simulink model "Grid_modelling_Thermal_V7_ALfix_sheddable"  (R2026a)
settings: Solver=ode45  StopTime=5000  MaxStep=0.01
libraries: sl_discontinuities x10, slpidlib x10, simulink x10
(part 2 of 3)

== system Grid_modelling_Thermal_V7_ALfix_sheddable/DAB_Model_HK ==
  phase_shift : Inport
  v_left : Inport  Port=2
  v_right : Inport  Port=3
  1/2*pi*fs : Gain  Gain=1 / (2*pi*10e3)
  1/Lk : Gain  Gain=1 / 340e-6
  Abs : Abs  SaturateOnIntegerOverflow=off
  Add Constant : Bias  Bias=1  SaturateOnIntegerOverflow=off
  Constant : Constant  Value=10
  DAB_Thermal_Model : Subsystem
  Divide : Product  Inputs=*/
  Divide1 : Product  Inputs=*/
  Gain : Gain  Gain=-1/pi
  Gain1 : Gain  Gain=-1
  Max : MinMax  Function=max  Inputs=2
  Max1 : MinMax  Function=max  Inputs=2
  Product : Product
  Product1 : Product  Inputs=3
  Saturation : Saturate  UpperLimit=pi/2  LowerLimit=-pi/2
  Saturation Dynamic : sl_discontinuities/Saturation Dynamic  OutMin=[]  OutMax=[]  OutDataTypeStr=Inherit: Same as second input  OutDataType=fixdt(1, 16)  OutScaling=2^-10  DoSatur=off
  V7DERLOG_V7DER_HK : ToWorkspace  VariableName=V7DER_HK  SaveFormat=Timeseries  SampleTime=0.01
  V7LOG_V7PH_HK : ToWorkspace  VariableName=V7PH_HK  SaveFormat=Timeseries  SampleTime=0.01
  V7TJLOG_V7TJ_HK : ToWorkspace  VariableName=V7TJ_HK  SaveFormat=Timeseries  SampleTime=0.01
  deg_2_rad : Gain  Gain=pi / 180
  thermal_derater : Subsystem
  turns_ratio : Gain  Gain=24/15
  i_dab_i : Outport
  i_dab_j : Outport  Port=2
  dab_k : Outport  Port=3
  Temp_Junction : Outport  Port=4
  Temp_HeatSink : Outport  Port=5
  wires:
  Constant/1 -> Max/2, Max1/2
  Add Constant/1 -> Product1/2
  Divide/1 -> Gain1/1
  Max1/1 -> Divide1/2
  Gain1/1 -> i_dab_i/1
  Divide1/1 -> i_dab_j/1
  Saturation Dynamic/1 -> DAB_Thermal_Model/1(P_ij), Divide1/1, Divide/1
  Saturation/1 -> Product1/1, Abs/1
  1/2*pi*fs/1 -> 1/Lk/1
  phase_shift/1 -> deg_2_rad/1, V7LOG_V7PH_HK/1
  Gain/1 -> Add Constant/1
  1/Lk/1 -> dab_k/1, Product1/3
  Product/1 -> turns_ratio/1
  turns_ratio/1 -> 1/2*pi*fs/1
  Abs/1 -> Gain/1
  deg_2_rad/1 -> Saturation/1
  Max/1 -> Divide/2
  v_right/1 -> DAB_Thermal_Model/3(Vb), Product/2, Max1/1
  v_left/1 -> DAB_Thermal_Model/2(Va), Max/1, Product/1
  Product1/1 -> Saturation Dynamic/2  "P_ij"
  DAB_Thermal_Model/1(T_j) -> thermal_derater/1(Tj), Temp_Junction/1, V7TJLOG_V7TJ_HK/1
  DAB_Thermal_Model/2(T_h) -> Temp_HeatSink/1
  thermal_derater/1(derate_pos) -> Saturation Dynamic/1, V7DERLOG_V7DER_HK/1
  thermal_derater/2(derate_neg) -> Saturation Dynamic/3

== system Grid_modelling_Thermal_V7_ALfix_sheddable/DAB_Model_KL ==
  phase_shift : Inport
  v_left : Inport  Port=2
  v_right : Inport  Port=3
  1/2*pi*fs : Gain  Gain=1 / (2*pi*10e3)
  1/Lk : Gain  Gain=1 / 340e-6
  Abs : Abs  SaturateOnIntegerOverflow=off
  Add Constant : Bias  Bias=1  SaturateOnIntegerOverflow=off
  Constant : Constant  Value=10
  DAB_Thermal_Model : Subsystem
  Divide : Product  Inputs=*/
  Divide1 : Product  Inputs=*/
  Gain : Gain  Gain=-1/pi
  Gain1 : Gain  Gain=-1
  Max : MinMax  Function=max  Inputs=2
  Max1 : MinMax  Function=max  Inputs=2
  Product : Product
  Product1 : Product  Inputs=3
  Saturation : Saturate  UpperLimit=pi/2  LowerLimit=-pi/2
  Saturation Dynamic : sl_discontinuities/Saturation Dynamic  OutMin=[]  OutMax=[]  OutDataTypeStr=Inherit: Same as second input  OutDataType=fixdt(1, 16)  OutScaling=2^-10  DoSatur=off
  V7DERLOG_V7DER_KL : ToWorkspace  VariableName=V7DER_KL  SaveFormat=Timeseries  SampleTime=0.01
  V7LOG_V7PH_KL : ToWorkspace  VariableName=V7PH_KL  SaveFormat=Timeseries  SampleTime=0.01
  V7TJLOG_V7TJ_KL : ToWorkspace  VariableName=V7TJ_KL  SaveFormat=Timeseries  SampleTime=0.01
  deg_2_rad : Gain  Gain=pi / 180
  thermal_derater : Subsystem
  turns_ratio : Gain  Gain=24/15
  i_dab_i : Outport
  i_dab_j : Outport  Port=2
  dab_k : Outport  Port=3
  Temp_Junction : Outport  Port=4
  Temp_HeatSink : Outport  Port=5
  wires:
  Constant/1 -> Max/2, Max1/2
  Add Constant/1 -> Product1/2
  Divide/1 -> Gain1/1
  Max1/1 -> Divide1/2
  Gain1/1 -> i_dab_i/1
  Divide1/1 -> i_dab_j/1
  Saturation Dynamic/1 -> DAB_Thermal_Model/1(P_ij), Divide1/1, Divide/1
  Saturation/1 -> Product1/1, Abs/1
  1/2*pi*fs/1 -> 1/Lk/1
  phase_shift/1 -> deg_2_rad/1, V7LOG_V7PH_KL/1
  Gain/1 -> Add Constant/1
  1/Lk/1 -> dab_k/1, Product1/3
  Product/1 -> turns_ratio/1
  turns_ratio/1 -> 1/2*pi*fs/1
  Abs/1 -> Gain/1
  deg_2_rad/1 -> Saturation/1
  Max/1 -> Divide/2
  v_right/1 -> DAB_Thermal_Model/3(Vb), Product/2, Max1/1
  v_left/1 -> DAB_Thermal_Model/2(Va), Max/1, Product/1
  Product1/1 -> Saturation Dynamic/2  "P_ij"
  DAB_Thermal_Model/1(T_j) -> thermal_derater/1(Tj), Temp_Junction/1, V7TJLOG_V7TJ_KL/1
  DAB_Thermal_Model/2(T_h) -> Temp_HeatSink/1
  thermal_derater/1(derate_pos) -> Saturation Dynamic/1, V7DERLOG_V7DER_KL/1
  thermal_derater/2(derate_neg) -> Saturation Dynamic/3

== system Grid_modelling_Thermal_V7_ALfix_sheddable/source_bus_model_A ==
  Pload : Inport
  i_dab_1 : Inport  Port=2
  i_dab_2 : Inport  Port=3
  1/C_bus : Gain  Gain=1/0.01
  1/Rsrc_k : Gain  Gain=1/(0.32*1)
  Add : Sum  Inputs=+-++
  Bus_Bar_Thermal_Model : Subsystem
  Constant : Constant  Value=0
  Divide : Product  Inputs=*/
  Divide1 : Product  Inputs=*/
  I_max : Constant  Value=125
  Integrator : Integrator  InitialCondition=800  LimitOutput=on  LowerSaturationLimit=0
  Max : MinMax  Function=max  Inputs=2
  Max1 : MinMax  Function=max  Inputs=2
  Max2 : MinMax  Function=max  Inputs=2
  Min : MinMax  Inputs=2
  Min1 : MinMax  Inputs=2
  P_max : Constant  Value=100e3
  Product : Product
  Subtract : Sum  Inputs=+-
  V_th_k : Constant  Value=800
  div_by_zero_protect : Constant  Value=10
  div_by_zero_protect1 : Constant  Value=10
  V_bus : Outport
  Bus_Power : Outport  Port=2
  Temp_bus : Outport  Port=3
  wires:
  Max2/1 -> Divide1/2
  Divide/1 -> Min1/2  "i_pmax_k"
  1/Rsrc_k/1 -> Max/1  "i_th_k"
  Min/1 -> Min1/1  "i_lim_k"
  Subtract/1 -> 1/Rsrc_k/1
  Add/1 -> 1/C_bus/1
  1/C_bus/1 -> Integrator/1
  Integrator/1 -> Product/1, V_bus/1, Max2/1, Max1/1, Subtract/2
  Divide1/1 -> Add/2
  V_th_k/1 -> Subtract/1
  Pload/1 -> Divide1/1
  Constant/1 -> Max/2
  Max/1 -> Min/1
  i_dab_1/1 -> Add/3
  I_max/1 -> Min/2
  Min1/1 -> Add/1, Bus_Bar_Thermal_Model/1(i_src_k), Product/2  "i_src_k"
  P_max/1 -> Divide/1
  Max1/1 -> Divide/2
  i_dab_2/1 -> Add/4
  div_by_zero_protect1/1 -> Max2/2
  div_by_zero_protect/1 -> Max1/2
  Product/1 -> Bus_Power/1
  Bus_Bar_Thermal_Model/1(T_bus) -> Temp_bus/1

== system Grid_modelling_Thermal_V7_ALfix_sheddable/source_bus_model_B ==
  Pload : Inport
  i_dab_1 : Inport  Port=2
  i_dab_2 : Inport  Port=3
  1/C_bus : Gain  Gain=1/0.01
  Add : Sum  Inputs=+-++
  Bus_Bar_Thermal_Model : Subsystem
  Constant : Constant  Value=0
  Divide : Product  Inputs=*/
  Divide1 : Product  Inputs=*/
  I_max : Constant  Value=125
  Integrator : Integrator  InitialCondition=800  LimitOutput=on  LowerSaturationLimit=0
  Max : MinMax  Function=max  Inputs=2
  Max1 : MinMax  Function=max  Inputs=2
  Max2 : MinMax  Function=max  Inputs=2
  Min : MinMax  Inputs=2
  Min1 : MinMax  Inputs=2
  P_max : Constant  Value=100e3
  Product : Product
  Product1 : Product
  Step : Step  Time=1000  InitialValue=1 / (0.32*1)  FinalValue=1 / (0.32*1)  SampleTime=0
  Subtract : Sum  Inputs=+-
  V_th_k : Constant  Value=800
  div_by_zero_protect : Constant  Value=10
  div_by_zero_protect1 : Constant  Value=10
  V_bus : Outport
  Bus_Power : Outport  Port=2
  Temp_bus : Outport  Port=3
  wires:
  Max2/1 -> Divide1/2
  Divide/1 -> Min1/2  "i_pmax_k"
  Product1/1 -> Max/1  "i_th_k"
  Min/1 -> Min1/1  "i_lim_k"
  Subtract/1 -> Product1/2
  Add/1 -> 1/C_bus/1
  1/C_bus/1 -> Integrator/1
  Divide1/1 -> Add/2
  V_th_k/1 -> Subtract/1
  Pload/1 -> Divide1/1
  Constant/1 -> Max/2
  Max/1 -> Min/1
  i_dab_1/1 -> Add/3
  I_max/1 -> Min/2
  P_max/1 -> Divide/1
  Max1/1 -> Divide/2
  i_dab_2/1 -> Add/4
  div_by_zero_protect1/1 -> Max2/2
  div_by_zero_protect/1 -> Max1/2
  Integrator/1 -> Product/1, V_bus/1, Max2/1, Max1/1, Subtract/2
  Product/1 -> Bus_Power/1
  Min1/1 -> Bus_Bar_Thermal_Model/1(i_src_k), Product/2, Add/1  "i_src_k"
  Bus_Bar_Thermal_Model/1(T_bus) -> Temp_bus/1
  Step/1 -> Product1/1

== system Grid_modelling_Thermal_V7_ALfix_sheddable/source_bus_model_C ==
  Pload : Inport
  i_dab_1 : Inport  Port=2
  i_dab_2 : Inport  Port=3
  1/C_bus : Gain  Gain=1/0.01
  Add : Sum  Inputs=+-++
  Bus_Bar_Thermal_Model : Subsystem
  Constant : Constant  Value=0
  Divide : Product  Inputs=*/
  Divide1 : Product  Inputs=*/
  I_max : Constant  Value=125
  Integrator : Integrator  InitialCondition=800  LimitOutput=on  LowerSaturationLimit=0
  Max : MinMax  Function=max  Inputs=2
  Max1 : MinMax  Function=max  Inputs=2
  Max2 : MinMax  Function=max  Inputs=2
  Min : MinMax  Inputs=2
  Min1 : MinMax  Inputs=2
  P_max : Constant  Value=100e3
  Product : Product
  Product1 : Product
  Step : Step  Time=2250  InitialValue=1 / (0.32*1)  FinalValue=1 / (0.32*1)  SampleTime=0
  Subtract : Sum  Inputs=+-
  V_th_k : Constant  Value=800
  div_by_zero_protect : Constant  Value=10
  div_by_zero_protect1 : Constant  Value=10
  V_bus : Outport
  Bus_Power : Outport  Port=2
  Temp_bus : Outport  Port=3
  wires:
  Max2/1 -> Divide1/2
  Divide/1 -> Min1/2  "i_pmax_k"
  Product1/1 -> Max/1  "i_th_k"
  Min/1 -> Min1/1  "i_lim_k"
  Subtract/1 -> Product1/2
  Add/1 -> 1/C_bus/1
  1/C_bus/1 -> Integrator/1
  Divide1/1 -> Add/2
  V_th_k/1 -> Subtract/1
  Pload/1 -> Divide1/1
  Constant/1 -> Max/2
  Max/1 -> Min/1
  i_dab_1/1 -> Add/3
  I_max/1 -> Min/2
  P_max/1 -> Divide/1
  Max1/1 -> Divide/2
  i_dab_2/1 -> Add/4
  div_by_zero_protect1/1 -> Max2/2
  div_by_zero_protect/1 -> Max1/2
  Integrator/1 -> Product/1, V_bus/1, Max2/1, Max1/1, Subtract/2
  Product/1 -> Bus_Power/1
  Min1/1 -> Bus_Bar_Thermal_Model/1(i_src_k), Product/2, Add/1  "i_src_k"
  Bus_Bar_Thermal_Model/1(T_bus) -> Temp_bus/1
  Step/1 -> Product1/1

== system Grid_modelling_Thermal_V7_ALfix_sheddable/source_bus_model_D ==
  Pload : Inport
  i_dab_1 : Inport  Port=2
  i_dab_2 : Inport  Port=3
  1/C_bus : Gain  Gain=1/0.01
  1/Rsrc_k : Gain  Gain=1/(0.32*1)
  Add : Sum  Inputs=+-++
  Bus_Bar_Thermal_Model : Subsystem
  Constant : Constant  Value=0
  Divide : Product  Inputs=*/
  Divide1 : Product  Inputs=*/
  I_max : Constant  Value=125
  Integrator : Integrator  InitialCondition=800  LimitOutput=on  LowerSaturationLimit=0
  Max : MinMax  Function=max  Inputs=2
  Max1 : MinMax  Function=max  Inputs=2
  Max2 : MinMax  Function=max  Inputs=2
  Min : MinMax  Inputs=2
  Min1 : MinMax  Inputs=2
  P_max : Constant  Value=100e3
  Product : Product
  Subtract : Sum  Inputs=+-
  V_th_k : Constant  Value=800
  div_by_zero_protect : Constant  Value=10
  div_by_zero_protect1 : Constant  Value=10
  V_bus : Outport
  Bus_Power : Outport  Port=2
  Temp_bus : Outport  Port=3
  wires:
  Max2/1 -> Divide1/2
  Divide/1 -> Min1/2  "i_pmax_k"
  1/Rsrc_k/1 -> Max/1  "i_th_k"
  Min/1 -> Min1/1  "i_lim_k"
  Subtract/1 -> 1/Rsrc_k/1
  Add/1 -> 1/C_bus/1
  1/C_bus/1 -> Integrator/1
  Divide1/1 -> Add/2
  V_th_k/1 -> Subtract/1
  Pload/1 -> Divide1/1
  Constant/1 -> Max/2
  Max/1 -> Min/1
  i_dab_1/1 -> Add/3
  I_max/1 -> Min/2
  P_max/1 -> Divide/1
  Max1/1 -> Divide/2
  i_dab_2/1 -> Add/4
  div_by_zero_protect1/1 -> Max2/2
  div_by_zero_protect/1 -> Max1/2
  Integrator/1 -> Product/1, V_bus/1, Max2/1, Max1/1, Subtract/2
  Product/1 -> Bus_Power/1
  Min1/1 -> Bus_Bar_Thermal_Model/1(i_src_k), Product/2, Add/1  "i_src_k"
  Bus_Bar_Thermal_Model/1(T_bus) -> Temp_bus/1

== system Grid_modelling_Thermal_V7_ALfix_sheddable/source_bus_model_E ==
  Pload : Inport
  i_dab_1 : Inport  Port=2
  i_dab_2 : Inport  Port=3
  1/C_bus : Gain  Gain=1/0.01
  Add : Sum  Inputs=+-++
  Bus_Bar_Thermal_Model : Subsystem
  Constant : Constant  Value=0
  Divide : Product  Inputs=*/
  Divide1 : Product  Inputs=*/
  I_max : Constant  Value=125
  Integrator : Integrator  InitialCondition=800  LimitOutput=on  LowerSaturationLimit=0
  Max : MinMax  Function=max  Inputs=2
  Max1 : MinMax  Function=max  Inputs=2
  Max2 : MinMax  Function=max  Inputs=2
  Min : MinMax  Inputs=2
  Min1 : MinMax  Inputs=2
  P_max : Constant  Value=70e3
  Product : Product
  Product1 : Product
  Step : Step  Time=1500  InitialValue=1 / (0.32*1)  FinalValue=1 / (0.32*2)  SampleTime=0
  Subtract : Sum  Inputs=+-
  V_th_k : Constant  Value=800
  div_by_zero_protect : Constant  Value=10
  div_by_zero_protect1 : Constant  Value=10
  V_bus : Outport
  Bus_Power : Outport  Port=2
  Temp_bus : Outport  Port=3
  wires:
  Max2/1 -> Divide1/2
  Divide/1 -> Min1/2  "i_pmax_k"
  Product1/1 -> Max/1  "i_th_k"
  Min/1 -> Min1/1  "i_lim_k"
  Subtract/1 -> Product1/2
  Add/1 -> 1/C_bus/1
  1/C_bus/1 -> Integrator/1
  Divide1/1 -> Add/2
  V_th_k/1 -> Subtract/1
  Pload/1 -> Divide1/1
  Constant/1 -> Max/2
  Max/1 -> Min/1
  i_dab_1/1 -> Add/3
  I_max/1 -> Min/2
  P_max/1 -> Divide/1
  Max1/1 -> Divide/2
  i_dab_2/1 -> Add/4
  div_by_zero_protect1/1 -> Max2/2
  div_by_zero_protect/1 -> Max1/2
  Integrator/1 -> Product/1, V_bus/1, Max2/1, Max1/1, Subtract/2
  Product/1 -> Bus_Power/1
  Min1/1 -> Bus_Bar_Thermal_Model/1(i_src_k), Product/2, Add/1  "i_src_k"
  Bus_Bar_Thermal_Model/1(T_bus) -> Temp_bus/1
  Step/1 -> Product1/1

== system Grid_modelling_Thermal_V7_ALfix_sheddable/source_bus_model_F ==
  Pload : Inport
  i_dab_1 : Inport  Port=2
  i_dab_2 : Inport  Port=3
  1/C_bus : Gain  Gain=1/0.01
  Add : Sum  Inputs=+-++
  Bus_Bar_Thermal_Model : Subsystem
  Constant : Constant  Value=0
  Divide : Product  Inputs=*/
  Divide1 : Product  Inputs=*/
  I_max : Constant  Value=125
  Integrator : Integrator  InitialCondition=800  LimitOutput=on  LowerSaturationLimit=0
  Max : MinMax  Function=max  Inputs=2
  Max1 : MinMax  Function=max  Inputs=2
  Max2 : MinMax  Function=max  Inputs=2
  Min : MinMax  Inputs=2
  Min1 : MinMax  Inputs=2
  P_max : Constant  Value=70e3
  Product : Product
  Product1 : Product
  Step : Step  Time=1250  InitialValue=1 / (0.32*1)  FinalValue=1 / (0.32*2)  SampleTime=0
  Subtract : Sum  Inputs=+-
  V_th_k : Constant  Value=800
  div_by_zero_protect : Constant  Value=10
  div_by_zero_protect1 : Constant  Value=10
  V_bus : Outport
  Bus_Power : Outport  Port=2
  Temp_bus : Outport  Port=3
  wires:
  Max2/1 -> Divide1/2
  Divide/1 -> Min1/2  "i_pmax_k"
  Product1/1 -> Max/1  "i_th_k"
  Min/1 -> Min1/1  "i_lim_k"
  Subtract/1 -> Product1/2
  Add/1 -> 1/C_bus/1
  1/C_bus/1 -> Integrator/1
  Divide1/1 -> Add/2
  V_th_k/1 -> Subtract/1
  Pload/1 -> Divide1/1
  Constant/1 -> Max/2
  Max/1 -> Min/1
  i_dab_1/1 -> Add/3
  I_max/1 -> Min/2
  P_max/1 -> Divide/1
  Max1/1 -> Divide/2
  i_dab_2/1 -> Add/4
  div_by_zero_protect1/1 -> Max2/2
  div_by_zero_protect/1 -> Max1/2
  Integrator/1 -> Product/1, V_bus/1, Max2/1, Max1/1, Subtract/2
  Product/1 -> Bus_Power/1
  Min1/1 -> Bus_Bar_Thermal_Model/1(i_src_k), Product/2, Add/1  "i_src_k"
  Bus_Bar_Thermal_Model/1(T_bus) -> Temp_bus/1
  Step/1 -> Product1/1

== system Grid_modelling_Thermal_V7_ALfix_sheddable/source_bus_model_G ==
  Pload : Inport
  i_dab_1 : Inport  Port=2
  i_dab_2 : Inport  Port=3
  1/C_bus : Gain  Gain=1/0.01
  1/Rsrc_k : Gain  Gain=1/(0.32*1)
  Add : Sum  Inputs=+-++
  Bus_Bar_Thermal_Model : Subsystem
  Constant : Constant  Value=0
  Divide : Product  Inputs=*/
  Divide1 : Product  Inputs=*/
  I_max : Constant  Value=125
  Integrator : Integrator  InitialCondition=800  LimitOutput=on  LowerSaturationLimit=0
  Max : MinMax  Function=max  Inputs=2
  Max1 : MinMax  Function=max  Inputs=2
  Max2 : MinMax  Function=max  Inputs=2
  Min : MinMax  Inputs=2
  Min1 : MinMax  Inputs=2
  P_max : Constant  Value=100e3
  Product : Product
  Subtract : Sum  Inputs=+-
  V_th_k : Constant  Value=800
  div_by_zero_protect : Constant  Value=10
  div_by_zero_protect1 : Constant  Value=10
  V_bus : Outport
  Bus_Power : Outport  Port=2
  Temp_bus : Outport  Port=3
  wires:
  Max2/1 -> Divide1/2
  Divide/1 -> Min1/2  "i_pmax_k"
  1/Rsrc_k/1 -> Max/1  "i_th_k"
  Min/1 -> Min1/1  "i_lim_k"
  Subtract/1 -> 1/Rsrc_k/1
  Add/1 -> 1/C_bus/1
  1/C_bus/1 -> Integrator/1
  Divide1/1 -> Add/2
  V_th_k/1 -> Subtract/1
  Pload/1 -> Divide1/1
  Constant/1 -> Max/2
  Max/1 -> Min/1
  i_dab_1/1 -> Add/3
  I_max/1 -> Min/2
  P_max/1 -> Divide/1
  Max1/1 -> Divide/2
  i_dab_2/1 -> Add/4
  div_by_zero_protect1/1 -> Max2/2
  div_by_zero_protect/1 -> Max1/2
  Integrator/1 -> Product/1, V_bus/1, Max2/1, Max1/1, Subtract/2
  Product/1 -> Bus_Power/1
  Min1/1 -> Bus_Bar_Thermal_Model/1(i_src_k), Product/2, Add/1  "i_src_k"
  Bus_Bar_Thermal_Model/1(T_bus) -> Temp_bus/1

== system Grid_modelling_Thermal_V7_ALfix_sheddable/source_bus_model_H ==
  Pload : Inport
  i_dab_1 : Inport  Port=2
  i_dab_2 : Inport  Port=3
  1/C_bus : Gain  Gain=1/0.01
  1/Rsrc_k : Gain  Gain=1/(0.32*1)
  Add : Sum  Inputs=+-++
  Bus_Bar_Thermal_Model : Subsystem
  Constant : Constant  Value=0
  Divide : Product  Inputs=*/
  Divide1 : Product  Inputs=*/
  I_max : Constant  Value=125
  Integrator : Integrator  InitialCondition=800  LimitOutput=on  LowerSaturationLimit=0
  Max : MinMax  Function=max  Inputs=2
  Max1 : MinMax  Function=max  Inputs=2
  Max2 : MinMax  Function=max  Inputs=2
  Min : MinMax  Inputs=2
  Min1 : MinMax  Inputs=2
  P_max : Constant  Value=100e3
  Product : Product
  Subtract : Sum  Inputs=+-
  V_th_k : Constant  Value=800
  div_by_zero_protect : Constant  Value=10
  div_by_zero_protect1 : Constant  Value=10
  V_bus : Outport
  Bus_Power : Outport  Port=2
  Temp_bus : Outport  Port=3
  wires:
  Max2/1 -> Divide1/2
  Divide/1 -> Min1/2  "i_pmax_k"
  1/Rsrc_k/1 -> Max/1  "i_th_k"
  Min/1 -> Min1/1  "i_lim_k"
  Subtract/1 -> 1/Rsrc_k/1
  Add/1 -> 1/C_bus/1
  1/C_bus/1 -> Integrator/1
  Divide1/1 -> Add/2
  V_th_k/1 -> Subtract/1
  Pload/1 -> Divide1/1
  Constant/1 -> Max/2
  Max/1 -> Min/1
  i_dab_1/1 -> Add/3
  I_max/1 -> Min/2
  P_max/1 -> Divide/1
  Max1/1 -> Divide/2
  i_dab_2/1 -> Add/4
  div_by_zero_protect1/1 -> Max2/2
  div_by_zero_protect/1 -> Max1/2
  Integrator/1 -> Product/1, V_bus/1, Max2/1, Max1/1, Subtract/2
  Product/1 -> Bus_Power/1
  Min1/1 -> Bus_Bar_Thermal_Model/1(i_src_k), Product/2, Add/1  "i_src_k"
  Bus_Bar_Thermal_Model/1(T_bus) -> Temp_bus/1

== system Grid_modelling_Thermal_V7_ALfix_sheddable/source_bus_model_K ==
  Pload : Inport
  i_dab_1 : Inport  Port=2
  i_dab_2 : Inport  Port=3
  1/C_bus : Gain  Gain=1/0.01
  1/Rsrc_k : Gain  Gain=1/(0.32*1)
  Add : Sum  Inputs=+-++
  Bus_Bar_Thermal_Model : Subsystem
  Constant : Constant  Value=0
  Divide : Product  Inputs=*/
  Divide1 : Product  Inputs=*/
  I_max : Constant  Value=125
  Integrator : Integrator  InitialCondition=800  LimitOutput=on  LowerSaturationLimit=0
  Max : MinMax  Function=max  Inputs=2
  Max1 : MinMax  Function=max  Inputs=2
  Max2 : MinMax  Function=max  Inputs=2
  Min : MinMax  Inputs=2
  Min1 : MinMax  Inputs=2
  P_max : Constant  Value=100e3
  Product : Product
  Subtract : Sum  Inputs=+-
  V_th_k : Constant  Value=800
  div_by_zero_protect : Constant  Value=10
  div_by_zero_protect1 : Constant  Value=10
  V_bus : Outport
  Bus_Power : Outport  Port=2
  Temp_bus : Outport  Port=3
  wires:
  Max2/1 -> Divide1/2
  Divide/1 -> Min1/2  "i_pmax_k"
  1/Rsrc_k/1 -> Max/1  "i_th_k"
  Min/1 -> Min1/1  "i_lim_k"
  Subtract/1 -> 1/Rsrc_k/1
  Add/1 -> 1/C_bus/1
  1/C_bus/1 -> Integrator/1
  Divide1/1 -> Add/2
  V_th_k/1 -> Subtract/1
  Pload/1 -> Divide1/1
  Constant/1 -> Max/2
  Max/1 -> Min/1
  i_dab_1/1 -> Add/3
  I_max/1 -> Min/2
  P_max/1 -> Divide/1
  Max1/1 -> Divide/2
  i_dab_2/1 -> Add/4
  div_by_zero_protect1/1 -> Max2/2
  div_by_zero_protect/1 -> Max1/2
  Integrator/1 -> Product/1, V_bus/1, Max2/1, Max1/1, Subtract/2
  Product/1 -> Bus_Power/1
  Min1/1 -> Bus_Bar_Thermal_Model/1(i_src_k), Product/2, Add/1  "i_src_k"
  Bus_Bar_Thermal_Model/1(T_bus) -> Temp_bus/1

== system Grid_modelling_Thermal_V7_ALfix_sheddable/source_bus_model_L ==
  Pload : Inport
  i_dab_1 : Inport  Port=2
  i_dab_2 : Inport  Port=3
  1/C_bus : Gain  Gain=1/0.01
  1/Rsrc_k : Gain  Gain=1/(0.32*1)
  Add : Sum  Inputs=+-++
  Bus_Bar_Thermal_Model : Subsystem
  Constant : Constant  Value=0
  Divide : Product  Inputs=*/
  Divide1 : Product  Inputs=*/
  I_max : Constant  Value=125
  Integrator : Integrator  InitialCondition=800  LimitOutput=on  LowerSaturationLimit=0
  Max : MinMax  Function=max  Inputs=2
  Max1 : MinMax  Function=max  Inputs=2
  Max2 : MinMax  Function=max  Inputs=2
  Min : MinMax  Inputs=2
  Min1 : MinMax  Inputs=2
  P_max : Constant  Value=100e3
  Product : Product
  Subtract : Sum  Inputs=+-
  V_th_k : Constant  Value=800
  div_by_zero_protect : Constant  Value=10
  div_by_zero_protect1 : Constant  Value=10
  V_bus : Outport
  Bus_Power : Outport  Port=2
  Temp_bus : Outport  Port=3
  wires:
  Max2/1 -> Divide1/2
  Divide/1 -> Min1/2  "i_pmax_k"
  1/Rsrc_k/1 -> Max/1  "i_th_k"
  Min/1 -> Min1/1  "i_lim_k"
  Subtract/1 -> 1/Rsrc_k/1
  Add/1 -> 1/C_bus/1
  1/C_bus/1 -> Integrator/1
  Divide1/1 -> Add/2
  V_th_k/1 -> Subtract/1
  Pload/1 -> Divide1/1
  Constant/1 -> Max/2
  Max/1 -> Min/1
  i_dab_1/1 -> Add/3
  I_max/1 -> Min/2
  P_max/1 -> Divide/1
  Max1/1 -> Divide/2
  i_dab_2/1 -> Add/4
  div_by_zero_protect1/1 -> Max2/2
  div_by_zero_protect/1 -> Max1/2
  Integrator/1 -> Product/1, V_bus/1, Max2/1, Max1/1, Subtract/2
  Product/1 -> Bus_Power/1
  Min1/1 -> Bus_Bar_Thermal_Model/1(i_src_k), Product/2, Add/1  "i_src_k"
  Bus_Bar_Thermal_Model/1(T_bus) -> Temp_bus/1

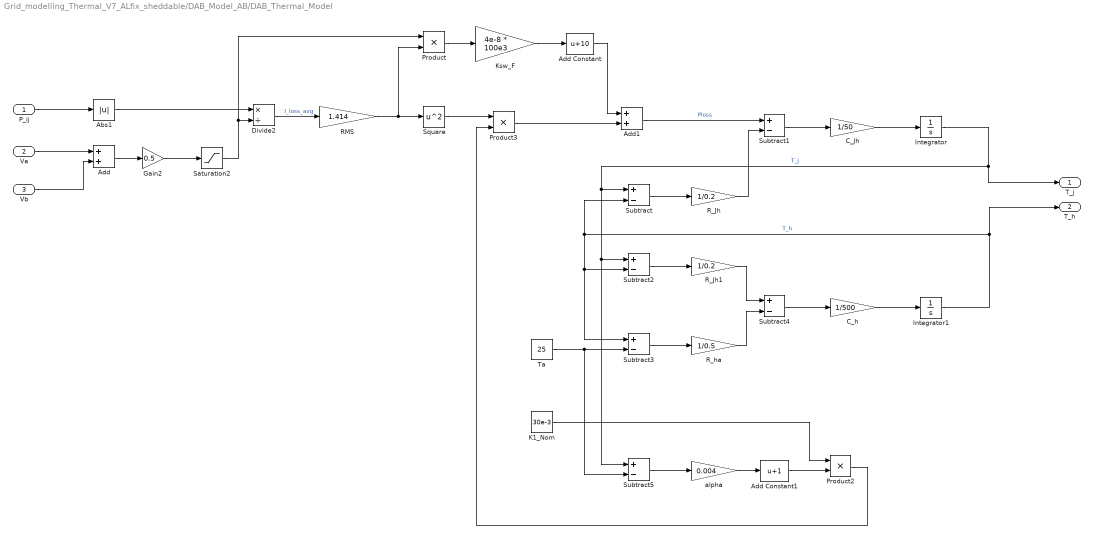
== system Grid_modelling_Thermal_V7_ALfix_sheddable/DAB_Model_AB/DAB_Thermal_Model ==
  P_ij : Inport
  Va : Inport  Port=2
  Vb : Inport  Port=3
  Abs1 : Abs  SaturateOnIntegerOverflow=off
  Add : Sum
  Add Constant : Bias  Bias=10  SaturateOnIntegerOverflow=off
  Add Constant1 : Bias  Bias=1  SaturateOnIntegerOverflow=off
  Add1 : Sum
  C_Jh : Gain  Gain=1/50
  C_h : Gain  Gain=1/500
  Divide2 : Product  Inputs=*/
  Gain2 : Gain  Gain=0.5
  Integrator : Integrator  InitialCondition=25
  Integrator1 : Integrator  InitialCondition=25
  K1_Nom : Constant  Value=30e-3
  Ksw_F : Gain  Gain=4e-8 * 100e3
  Product : Product
  Product2 : Product
  Product3 : Product
  RMS : Gain  Gain=1.414
  R_Jh : Gain  Gain=1/0.2
  R_Jh1 : Gain  Gain=1/0.2
  R_ha : Gain  Gain=1/0.5
  Saturation2 : Saturate  UpperLimit=inf  LowerLimit=1e-3
  Square : Math  Operator=square
  Subtract{,1..5} (6 alike) : Sum  Inputs=+-
  Ta : Constant  Value=25
  alpha : Gain  Gain=0.004
  T_j : Outport
  T_h : Outport  Port=2
  wires:
  Integrator/1 -> T_j/1, Subtract5/1, Subtract2/1, Subtract/1  "T_j"
  Add1/1 -> Subtract1/1  "Ploss"
  R_ha/1 -> Subtract4/2
  Gain2/1 -> Saturation2/1
  Va/1 -> Add/1
  Integrator1/1 -> T_h/1, Subtract/2, Subtract3/1, Subtract2/2  "T_h"
  R_Jh/1 -> Subtract1/2
  Add/1 -> Gain2/1
  Subtract5/1 -> alpha/1
  Subtract1/1 -> C_Jh/1
  C_h/1 -> Integrator1/1
  Divide2/1 -> RMS/1  "I_loss_avg"
  Product3/1 -> Add1/2
  P_ij/1 -> Abs1/1
  Subtract2/1 -> R_Jh1/1
  alpha/1 -> Add Constant1/1
  Product2/1 -> Product3/2
  C_Jh/1 -> Integrator/1
  Ta/1 -> Subtract5/2, Subtract3/2
  Saturation2/1 -> Product/1, Divide2/2
  R_Jh1/1 -> Subtract4/1
  Subtract/1 -> R_Jh/1
  Abs1/1 -> Divide2/1
  Subtract4/1 -> C_h/1
  Subtract3/1 -> R_ha/1
  Add Constant1/1 -> Product2/2
  Vb/1 -> Add/2
  K1_Nom/1 -> Product2/1
  Square/1 -> Product3/1
  RMS/1 -> Product/2, Square/1
  Product/1 -> Ksw_F/1
  Ksw_F/1 -> Add Constant/1
  Add Constant/1 -> Add1/1

== system Grid_modelling_Thermal_V7_ALfix_sheddable/DAB_Model_AB/thermal_derater ==
  Tj : Inport
  Gain : Gain  Gain=-1
  Gain2 : Gain  Gain=100e3
  If : If  IfExpression=u1 < 125  ElseIfExpressions=u1 > 125 & u1 < 175, u1 > 175  ShowElse=off
  If Action Subsystem : Subsystem  TreatAsAtomicUnit=on
  If Action Subsystem1 : Subsystem  TreatAsAtomicUnit=on
  If Action Subsystem2 : Subsystem  TreatAsAtomicUnit=on
  Merge : Merge  Inputs=3
  Saturation2 : Saturate  UpperLimit=1  LowerLimit=0
  Scope : Scope
      settings: ActiveDisplayYMinimum=0.36463  ActiveDisplayYMaximum=1.0706  DataLoggingVariableName=ScopeData2
  derate_pos : Outport
  derate_neg : Outport  Port=2
  wires:
  If/1 -> If Action Subsystem/Action
  Tj/1 -> If/1, If Action Subsystem1/1(Tj)
  If/3 -> If Action Subsystem2/Action
  If Action Subsystem2/1(Out1) -> Merge/3
  If Action Subsystem1/1(Out1) -> Merge/2
  Merge/1 -> Saturation2/1
  If Action Subsystem/1(Out1) -> Merge/1
  Gain2/1 -> derate_pos/1, Gain/1
  Saturation2/1 -> Scope/1, Gain2/1  "DAB_AB_derate_factor"
  Gain/1 -> derate_neg/1
  If/2 -> If Action Subsystem1/Action

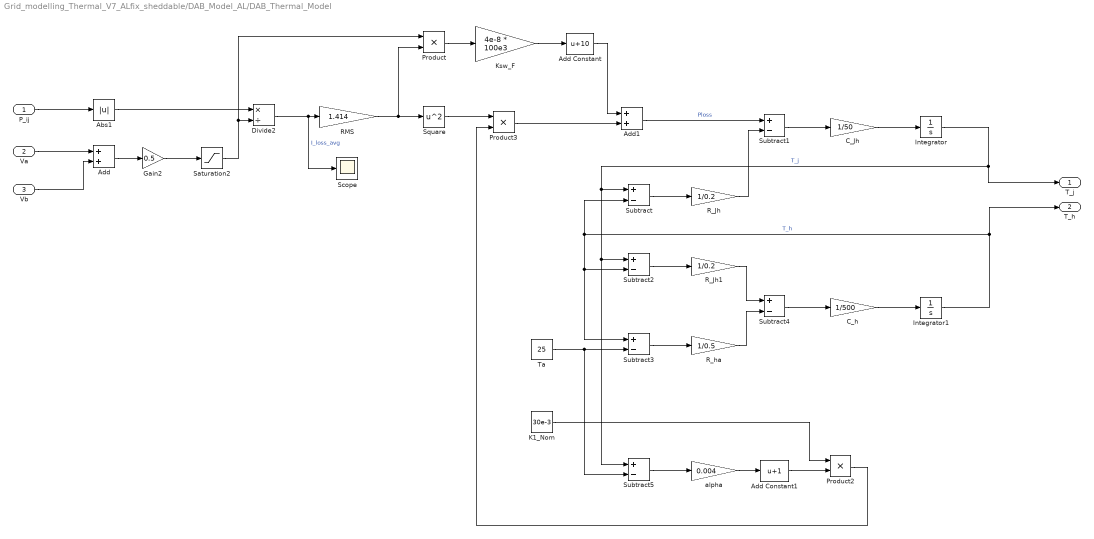
== system Grid_modelling_Thermal_V7_ALfix_sheddable/DAB_Model_AL/DAB_Thermal_Model ==
  P_ij : Inport
  Va : Inport  Port=2
  Vb : Inport  Port=3
  Abs1 : Abs  SaturateOnIntegerOverflow=off
  Add : Sum
  Add Constant : Bias  Bias=10  SaturateOnIntegerOverflow=off
  Add Constant1 : Bias  Bias=1  SaturateOnIntegerOverflow=off
  Add1 : Sum
  C_Jh : Gain  Gain=1/50
  C_h : Gain  Gain=1/500
  Divide2 : Product  Inputs=*/
  Gain2 : Gain  Gain=0.5
  Integrator : Integrator  InitialCondition=25
  Integrator1 : Integrator  InitialCondition=25
  K1_Nom : Constant  Value=30e-3
  Ksw_F : Gain  Gain=4e-8 * 100e3
  Product : Product
  Product2 : Product
  Product3 : Product
  RMS : Gain  Gain=1.414
  R_Jh : Gain  Gain=1/0.2
  R_Jh1 : Gain  Gain=1/0.2
  R_ha : Gain  Gain=1/0.5
  Saturation2 : Saturate  UpperLimit=inf  LowerLimit=1e-3
  Scope : Scope
      settings: ActiveDisplayYMinimum=-2.45667  ActiveDisplayYMaximum=22.11007
  Square : Math  Operator=square
  Subtract{,1..5} (6 alike) : Sum  Inputs=+-
  Ta : Constant  Value=25
  alpha : Gain  Gain=0.004
  T_j : Outport
  T_h : Outport  Port=2
  wires:
  Integrator/1 -> T_j/1, Subtract5/1, Subtract2/1, Subtract/1  "T_j"
  Add1/1 -> Subtract1/1  "Ploss"
  R_ha/1 -> Subtract4/2
  Gain2/1 -> Saturation2/1
  Va/1 -> Add/1
  Integrator1/1 -> T_h/1, Subtract/2, Subtract3/1, Subtract2/2  "T_h"
  R_Jh/1 -> Subtract1/2
  Add/1 -> Gain2/1
  Subtract5/1 -> alpha/1
  Subtract1/1 -> C_Jh/1
  C_h/1 -> Integrator1/1
  Divide2/1 -> Scope/1, RMS/1  "I_loss_avg"
  Product3/1 -> Add1/2
  P_ij/1 -> Abs1/1
  Subtract2/1 -> R_Jh1/1
  alpha/1 -> Add Constant1/1
  Product2/1 -> Product3/2
  C_Jh/1 -> Integrator/1
  Ta/1 -> Subtract5/2, Subtract3/2
  Saturation2/1 -> Product/1, Divide2/2
  R_Jh1/1 -> Subtract4/1
  Subtract/1 -> R_Jh/1
  Abs1/1 -> Divide2/1
  Subtract4/1 -> C_h/1
  Subtract3/1 -> R_ha/1
  Add Constant1/1 -> Product2/2
  Vb/1 -> Add/2
  K1_Nom/1 -> Product2/1
  Square/1 -> Product3/1
  RMS/1 -> Product/2, Square/1
  Product/1 -> Ksw_F/1
  Ksw_F/1 -> Add Constant/1
  Add Constant/1 -> Add1/1

== system Grid_modelling_Thermal_V7_ALfix_sheddable/DAB_Model_AL/thermal_derater ==
  Tj : Inport
  Gain : Gain  Gain=-1
  Gain2 : Gain  Gain=100e3
  If : If  IfExpression=u1 < 125  ElseIfExpressions=u1 > 125 & u1 < 175, u1 > 175  ShowElse=off
  If Action Subsystem : Subsystem  TreatAsAtomicUnit=on
  If Action Subsystem1 : Subsystem  TreatAsAtomicUnit=on
  If Action Subsystem2 : Subsystem  TreatAsAtomicUnit=on
  Merge : Merge  Inputs=3
  Saturation2 : Saturate  UpperLimit=1  LowerLimit=0
  Scope : Scope
      settings: ActiveDisplayYMinimum=0.11245  ActiveDisplayYMaximum=1.09862  DataLoggingVariableName=ScopeData2
  derate_pos : Outport
  derate_neg : Outport  Port=2
  wires:
  If/1 -> If Action Subsystem/Action
  Tj/1 -> If/1, If Action Subsystem1/1(Tj)
  If/3 -> If Action Subsystem2/Action
  If/2 -> If Action Subsystem1/Action
  If Action Subsystem2/1(Out1) -> Merge/3
  If Action Subsystem1/1(Out1) -> Merge/2
  Merge/1 -> Saturation2/1
  If Action Subsystem/1(Out1) -> Merge/1
  Gain2/1 -> derate_pos/1, Gain/1
  Saturation2/1 -> Scope/1, Gain2/1  "DAB_AL_derate_factor"
  Gain/1 -> derate_neg/1

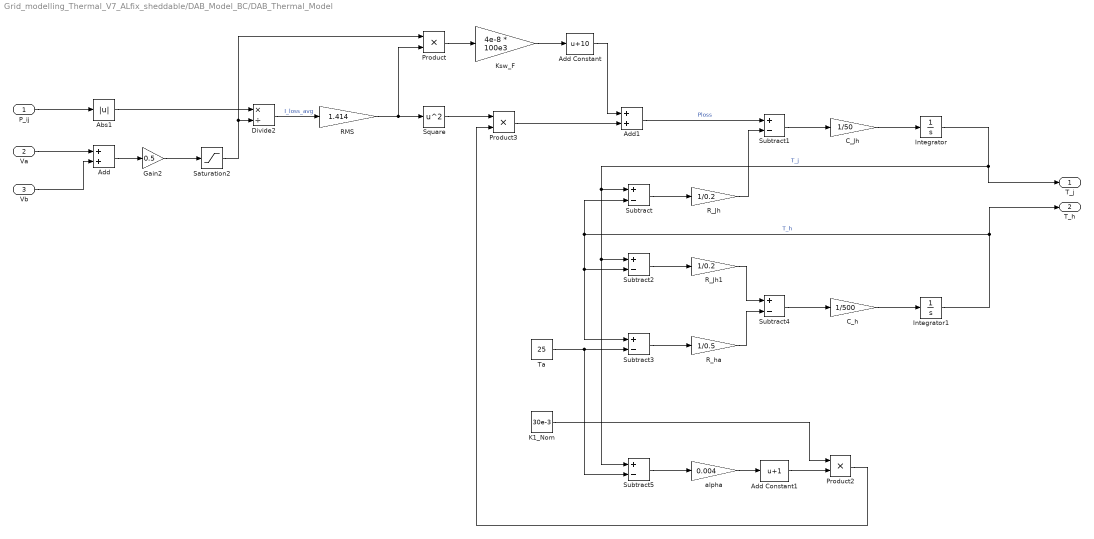
== system Grid_modelling_Thermal_V7_ALfix_sheddable/DAB_Model_BC/DAB_Thermal_Model ==
  P_ij : Inport
  Va : Inport  Port=2
  Vb : Inport  Port=3
  Abs1 : Abs  SaturateOnIntegerOverflow=off
  Add : Sum
  Add Constant : Bias  Bias=10  SaturateOnIntegerOverflow=off
  Add Constant1 : Bias  Bias=1  SaturateOnIntegerOverflow=off
  Add1 : Sum
  C_Jh : Gain  Gain=1/50
  C_h : Gain  Gain=1/500
  Divide2 : Product  Inputs=*/
  Gain2 : Gain  Gain=0.5
  Integrator : Integrator  InitialCondition=25
  Integrator1 : Integrator  InitialCondition=25
  K1_Nom : Constant  Value=30e-3
  Ksw_F : Gain  Gain=4e-8 * 100e3
  Product : Product
  Product2 : Product
  Product3 : Product
  RMS : Gain  Gain=1.414
  R_Jh : Gain  Gain=1/0.2
  R_Jh1 : Gain  Gain=1/0.2
  R_ha : Gain  Gain=1/0.5
  Saturation2 : Saturate  UpperLimit=inf  LowerLimit=1e-3
  Square : Math  Operator=square
  Subtract{,1..5} (6 alike) : Sum  Inputs=+-
  Ta : Constant  Value=25
  alpha : Gain  Gain=0.004
  T_j : Outport
  T_h : Outport  Port=2
  wires:
  Integrator/1 -> T_j/1, Subtract5/1, Subtract2/1, Subtract/1  "T_j"
  Add1/1 -> Subtract1/1  "Ploss"
  R_ha/1 -> Subtract4/2
  Gain2/1 -> Saturation2/1
  Va/1 -> Add/1
  Integrator1/1 -> T_h/1, Subtract/2, Subtract3/1, Subtract2/2  "T_h"
  R_Jh/1 -> Subtract1/2
  Add/1 -> Gain2/1
  Subtract5/1 -> alpha/1
  Subtract1/1 -> C_Jh/1
  C_h/1 -> Integrator1/1
  Divide2/1 -> RMS/1  "I_loss_avg"
  Product3/1 -> Add1/2
  P_ij/1 -> Abs1/1
  Subtract2/1 -> R_Jh1/1
  alpha/1 -> Add Constant1/1
  Product2/1 -> Product3/2
  C_Jh/1 -> Integrator/1
  Ta/1 -> Subtract5/2, Subtract3/2
  Saturation2/1 -> Product/1, Divide2/2
  R_Jh1/1 -> Subtract4/1
  Subtract/1 -> R_Jh/1
  Abs1/1 -> Divide2/1
  Subtract4/1 -> C_h/1
  Subtract3/1 -> R_ha/1
  Add Constant1/1 -> Product2/2
  Vb/1 -> Add/2
  K1_Nom/1 -> Product2/1
  Square/1 -> Product3/1
  RMS/1 -> Product/2, Square/1
  Product/1 -> Ksw_F/1
  Ksw_F/1 -> Add Constant/1
  Add Constant/1 -> Add1/1

== system Grid_modelling_Thermal_V7_ALfix_sheddable/DAB_Model_BC/thermal_derater ==
  Tj : Inport
  Gain : Gain  Gain=-1
  Gain2 : Gain  Gain=100e3
  If : If  IfExpression=u1 < 125  ElseIfExpressions=u1 > 125 & u1 < 175, u1 > 175  ShowElse=off
  If Action Subsystem : Subsystem  TreatAsAtomicUnit=on
  If Action Subsystem1 : Subsystem  TreatAsAtomicUnit=on
  If Action Subsystem2 : Subsystem  TreatAsAtomicUnit=on
  Merge : Merge  Inputs=3
  Saturation2 : Saturate  UpperLimit=1  LowerLimit=0
  Scope : Scope
      settings: ActiveDisplayYMinimum=0.62626  ActiveDisplayYMaximum=1.04153  DataLoggingVariableName=ScopeData2
  derate_pos : Outport
  derate_neg : Outport  Port=2
  wires:
  If/1 -> If Action Subsystem/Action
  Tj/1 -> If/1, If Action Subsystem1/1(Tj)
  If/3 -> If Action Subsystem2/Action
  If/2 -> If Action Subsystem1/Action
  If Action Subsystem2/1(Out1) -> Merge/3
  If Action Subsystem1/1(Out1) -> Merge/2
  Merge/1 -> Saturation2/1
  If Action Subsystem/1(Out1) -> Merge/1
  Gain2/1 -> derate_pos/1, Gain/1
  Saturation2/1 -> Scope/1, Gain2/1  "DAB_BC_derate_factor"
  Gain/1 -> derate_neg/1

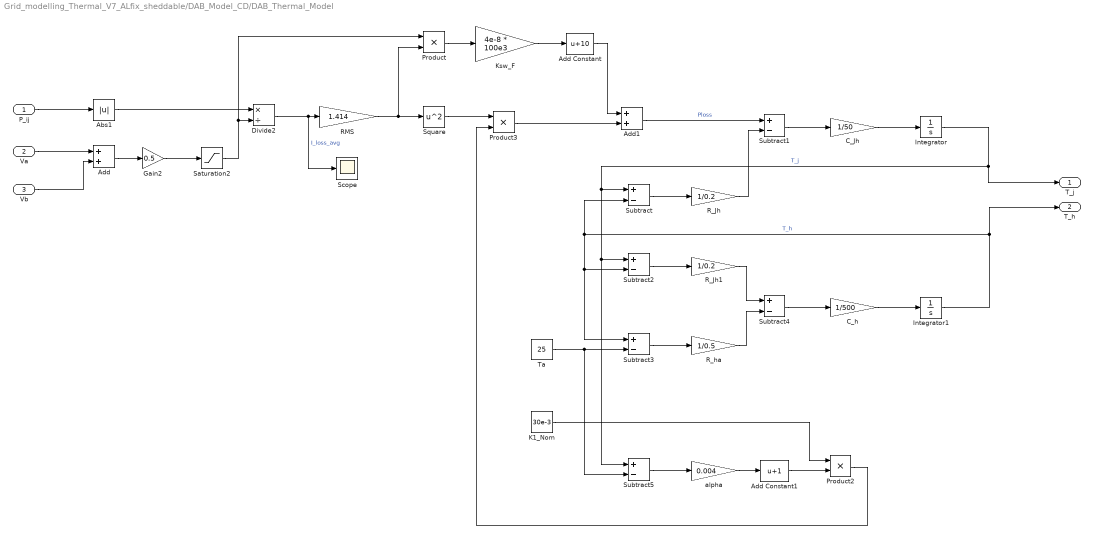
== system Grid_modelling_Thermal_V7_ALfix_sheddable/DAB_Model_CD/DAB_Thermal_Model ==
  P_ij : Inport
  Va : Inport  Port=2
  Vb : Inport  Port=3
  Abs1 : Abs  SaturateOnIntegerOverflow=off
  Add : Sum
  Add Constant : Bias  Bias=10  SaturateOnIntegerOverflow=off
  Add Constant1 : Bias  Bias=1  SaturateOnIntegerOverflow=off
  Add1 : Sum
  C_Jh : Gain  Gain=1/50
  C_h : Gain  Gain=1/500
  Divide2 : Product  Inputs=*/
  Gain2 : Gain  Gain=0.5
  Integrator : Integrator  InitialCondition=25
  Integrator1 : Integrator  InitialCondition=25
  K1_Nom : Constant  Value=30e-3
  Ksw_F : Gain  Gain=4e-8 * 100e3
  Product : Product
  Product2 : Product
  Product3 : Product
  RMS : Gain  Gain=1.414
  R_Jh : Gain  Gain=1/0.2
  R_Jh1 : Gain  Gain=1/0.2
  R_ha : Gain  Gain=1/0.5
  Saturation2 : Saturate  UpperLimit=inf  LowerLimit=1e-3
  Scope : Scope
      settings: ActiveDisplayYMinimum=-2.45667  ActiveDisplayYMaximum=22.11007
  Square : Math  Operator=square
  Subtract{,1..5} (6 alike) : Sum  Inputs=+-
  Ta : Constant  Value=25
  alpha : Gain  Gain=0.004
  T_j : Outport
  T_h : Outport  Port=2
  wires:
  Integrator/1 -> T_j/1, Subtract5/1, Subtract2/1, Subtract/1  "T_j"
  Add1/1 -> Subtract1/1  "Ploss"
  R_ha/1 -> Subtract4/2
  Gain2/1 -> Saturation2/1
  Va/1 -> Add/1
  Integrator1/1 -> T_h/1, Subtract/2, Subtract3/1, Subtract2/2  "T_h"
  R_Jh/1 -> Subtract1/2
  Add/1 -> Gain2/1
  Subtract5/1 -> alpha/1
  Subtract1/1 -> C_Jh/1
  C_h/1 -> Integrator1/1
  Divide2/1 -> Scope/1, RMS/1  "I_loss_avg"
  Product3/1 -> Add1/2
  P_ij/1 -> Abs1/1
  Subtract2/1 -> R_Jh1/1
  alpha/1 -> Add Constant1/1
  Product2/1 -> Product3/2
  C_Jh/1 -> Integrator/1
  Ta/1 -> Subtract5/2, Subtract3/2
  Saturation2/1 -> Product/1, Divide2/2
  R_Jh1/1 -> Subtract4/1
  Subtract/1 -> R_Jh/1
  Abs1/1 -> Divide2/1
  Subtract4/1 -> C_h/1
  Subtract3/1 -> R_ha/1
  Add Constant1/1 -> Product2/2
  Vb/1 -> Add/2
  K1_Nom/1 -> Product2/1
  Square/1 -> Product3/1
  RMS/1 -> Product/2, Square/1
  Product/1 -> Ksw_F/1
  Ksw_F/1 -> Add Constant/1
  Add Constant/1 -> Add1/1

== system Grid_modelling_Thermal_V7_ALfix_sheddable/DAB_Model_CD/thermal_derater ==
  Tj : Inport
  Gain : Gain  Gain=-1
  Gain2 : Gain  Gain=100e3
  If : If  IfExpression=u1 < 125  ElseIfExpressions=u1 > 125 & u1 < 175, u1 > 175  ShowElse=off
  If Action Subsystem : Subsystem  TreatAsAtomicUnit=on
  If Action Subsystem1 : Subsystem  TreatAsAtomicUnit=on
  If Action Subsystem2 : Subsystem  TreatAsAtomicUnit=on
  Merge : Merge  Inputs=3
  Saturation2 : Saturate  UpperLimit=1  LowerLimit=0
  Scope : Scope
      settings: ActiveDisplayYMinimum=0.06061  ActiveDisplayYMaximum=1.10438  DataLoggingVariableName=ScopeData2
  derate_pos : Outport
  derate_neg : Outport  Port=2
  wires:
  If/1 -> If Action Subsystem/Action
  Tj/1 -> If/1, If Action Subsystem1/1(Tj)
  If/3 -> If Action Subsystem2/Action
  If/2 -> If Action Subsystem1/Action
  If Action Subsystem2/1(Out1) -> Merge/3
  If Action Subsystem1/1(Out1) -> Merge/2
  Merge/1 -> Saturation2/1
  If Action Subsystem/1(Out1) -> Merge/1
  Gain2/1 -> derate_pos/1, Gain/1
  Saturation2/1 -> Scope/1, Gain2/1  "DAB_CD_derate_factor"
  Gain/1 -> derate_neg/1

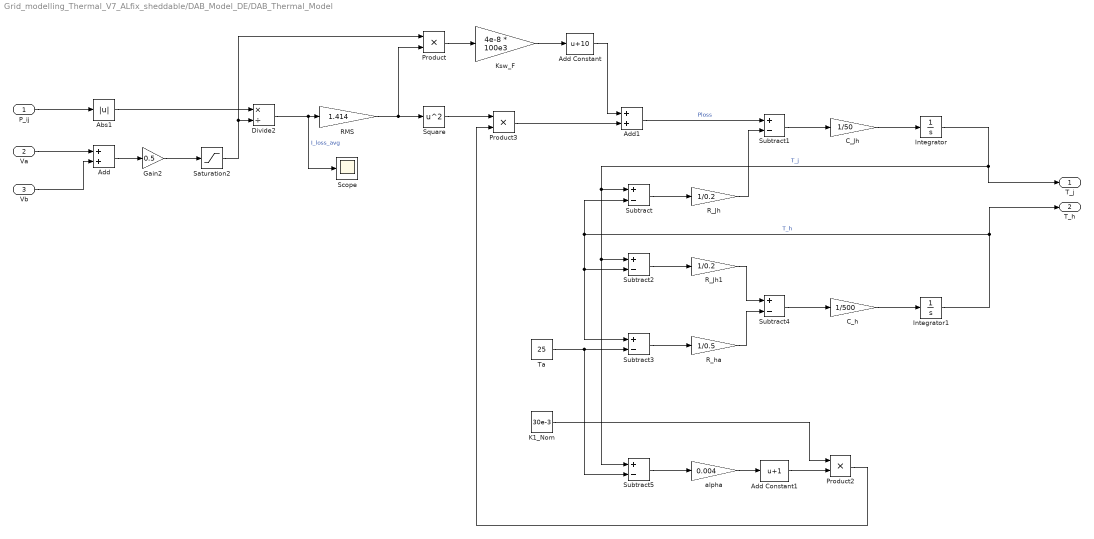
== system Grid_modelling_Thermal_V7_ALfix_sheddable/DAB_Model_DE/DAB_Thermal_Model ==
  P_ij : Inport
  Va : Inport  Port=2
  Vb : Inport  Port=3
  Abs1 : Abs  SaturateOnIntegerOverflow=off
  Add : Sum
  Add Constant : Bias  Bias=10  SaturateOnIntegerOverflow=off
  Add Constant1 : Bias  Bias=1  SaturateOnIntegerOverflow=off
  Add1 : Sum
  C_Jh : Gain  Gain=1/50
  C_h : Gain  Gain=1/500
  Divide2 : Product  Inputs=*/
  Gain2 : Gain  Gain=0.5
  Integrator : Integrator  InitialCondition=25
  Integrator1 : Integrator  InitialCondition=25
  K1_Nom : Constant  Value=30e-3
  Ksw_F : Gain  Gain=4e-8 * 100e3
  Product : Product
  Product2 : Product
  Product3 : Product
  RMS : Gain  Gain=1.414
  R_Jh : Gain  Gain=1/0.2
  R_Jh1 : Gain  Gain=1/0.2
  R_ha : Gain  Gain=1/0.5
  Saturation2 : Saturate  UpperLimit=inf  LowerLimit=1e-3
  Scope : Scope
      settings: ActiveDisplayYMinimum=-2.45667  ActiveDisplayYMaximum=22.11007
  Square : Math  Operator=square
  Subtract{,1..5} (6 alike) : Sum  Inputs=+-
  Ta : Constant  Value=25
  alpha : Gain  Gain=0.004
  T_j : Outport
  T_h : Outport  Port=2
  wires:
  Integrator/1 -> T_j/1, Subtract5/1, Subtract2/1, Subtract/1  "T_j"
  Add1/1 -> Subtract1/1  "Ploss"
  R_ha/1 -> Subtract4/2
  Gain2/1 -> Saturation2/1
  Va/1 -> Add/1
  Integrator1/1 -> T_h/1, Subtract/2, Subtract3/1, Subtract2/2  "T_h"
  R_Jh/1 -> Subtract1/2
  Add/1 -> Gain2/1
  Subtract5/1 -> alpha/1
  Subtract1/1 -> C_Jh/1
  C_h/1 -> Integrator1/1
  Divide2/1 -> Scope/1, RMS/1  "I_loss_avg"
  Product3/1 -> Add1/2
  P_ij/1 -> Abs1/1
  Subtract2/1 -> R_Jh1/1
  alpha/1 -> Add Constant1/1
  Product2/1 -> Product3/2
  C_Jh/1 -> Integrator/1
  Ta/1 -> Subtract5/2, Subtract3/2
  Saturation2/1 -> Product/1, Divide2/2
  R_Jh1/1 -> Subtract4/1
  Subtract/1 -> R_Jh/1
  Abs1/1 -> Divide2/1
  Subtract4/1 -> C_h/1
  Subtract3/1 -> R_ha/1
  Add Constant1/1 -> Product2/2
  Vb/1 -> Add/2
  K1_Nom/1 -> Product2/1
  Square/1 -> Product3/1
  RMS/1 -> Product/2, Square/1
  Product/1 -> Ksw_F/1
  Ksw_F/1 -> Add Constant/1
  Add Constant/1 -> Add1/1

== system Grid_modelling_Thermal_V7_ALfix_sheddable/DAB_Model_DE/thermal_derater ==
  Tj : Inport
  Gain : Gain  Gain=-1
  Gain2 : Gain  Gain=100e3
  If : If  IfExpression=u1 < 125  ElseIfExpressions=u1 > 125 & u1 < 175, u1 > 175  ShowElse=off
  If Action Subsystem : Subsystem  TreatAsAtomicUnit=on
  If Action Subsystem1 : Subsystem  TreatAsAtomicUnit=on
  If Action Subsystem2 : Subsystem  TreatAsAtomicUnit=on
  Merge : Merge  Inputs=3
  Saturation2 : Saturate  UpperLimit=1  LowerLimit=0
  Scope : Scope
      settings: ActiveDisplayYMinimum=0.11302  ActiveDisplayYMaximum=1.09855  DataLoggingVariableName=ScopeData2
  derate_pos : Outport
  derate_neg : Outport  Port=2
  wires:
  If/1 -> If Action Subsystem/Action
  Tj/1 -> If/1, If Action Subsystem1/1(Tj)
  If/3 -> If Action Subsystem2/Action
  If/2 -> If Action Subsystem1/Action
  If Action Subsystem2/1(Out1) -> Merge/3
  If Action Subsystem1/1(Out1) -> Merge/2
  Merge/1 -> Saturation2/1
  If Action Subsystem/1(Out1) -> Merge/1
  Gain2/1 -> derate_pos/1, Gain/1
  Saturation2/1 -> Scope/1, Gain2/1  "DAB_DE_derate_factor"
  Gain/1 -> derate_neg/1

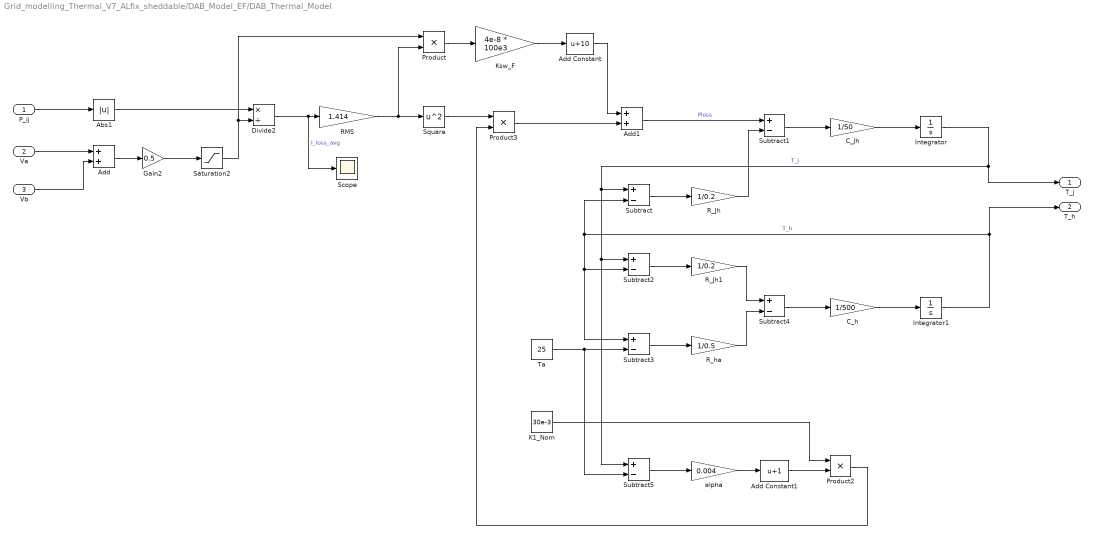
== system Grid_modelling_Thermal_V7_ALfix_sheddable/DAB_Model_EF/DAB_Thermal_Model ==
  P_ij : Inport
  Va : Inport  Port=2
  Vb : Inport  Port=3
  Abs1 : Abs  SaturateOnIntegerOverflow=off
  Add : Sum
  Add Constant : Bias  Bias=10  SaturateOnIntegerOverflow=off
  Add Constant1 : Bias  Bias=1  SaturateOnIntegerOverflow=off
  Add1 : Sum
  C_Jh : Gain  Gain=1/50
  C_h : Gain  Gain=1/500
  Divide2 : Product  Inputs=*/
  Gain2 : Gain  Gain=0.5
  Integrator : Integrator  InitialCondition=25
  Integrator1 : Integrator  InitialCondition=25
  K1_Nom : Constant  Value=30e-3
  Ksw_F : Gain  Gain=4e-8 * 100e3
  Product : Product
  Product2 : Product
  Product3 : Product
  RMS : Gain  Gain=1.414
  R_Jh : Gain  Gain=1/0.2
  R_Jh1 : Gain  Gain=1/0.2
  R_ha : Gain  Gain=1/0.5
  Saturation2 : Saturate  UpperLimit=inf  LowerLimit=1e-3
  Scope : Scope
      settings: ActiveDisplayYMinimum=-2.45667  ActiveDisplayYMaximum=22.11007
  Square : Math  Operator=square
  Subtract{,1..5} (6 alike) : Sum  Inputs=+-
  Ta : Constant  Value=25
  alpha : Gain  Gain=0.004
  T_j : Outport
  T_h : Outport  Port=2
  wires:
  Integrator/1 -> T_j/1, Subtract5/1, Subtract2/1, Subtract/1  "T_j"
  Add1/1 -> Subtract1/1  "Ploss"
  R_ha/1 -> Subtract4/2
  Gain2/1 -> Saturation2/1
  Va/1 -> Add/1
  Integrator1/1 -> T_h/1, Subtract/2, Subtract3/1, Subtract2/2  "T_h"
  R_Jh/1 -> Subtract1/2
  Add/1 -> Gain2/1
  Subtract5/1 -> alpha/1
  Subtract1/1 -> C_Jh/1
  C_h/1 -> Integrator1/1
  Divide2/1 -> Scope/1, RMS/1  "I_loss_avg"
  Product3/1 -> Add1/2
  P_ij/1 -> Abs1/1
  Subtract2/1 -> R_Jh1/1
  alpha/1 -> Add Constant1/1
  Product2/1 -> Product3/2
  C_Jh/1 -> Integrator/1
  Ta/1 -> Subtract5/2, Subtract3/2
  Saturation2/1 -> Product/1, Divide2/2
  R_Jh1/1 -> Subtract4/1
  Subtract/1 -> R_Jh/1
  Abs1/1 -> Divide2/1
  Subtract4/1 -> C_h/1
  Subtract3/1 -> R_ha/1
  Add Constant1/1 -> Product2/2
  Vb/1 -> Add/2
  K1_Nom/1 -> Product2/1
  Square/1 -> Product3/1
  RMS/1 -> Product/2, Square/1
  Product/1 -> Ksw_F/1
  Ksw_F/1 -> Add Constant/1
  Add Constant/1 -> Add1/1

== system Grid_modelling_Thermal_V7_ALfix_sheddable/DAB_Model_EF/thermal_derater ==
  Tj : Inport
  Gain : Gain  Gain=-1
  Gain2 : Gain  Gain=100e3
  If : If  IfExpression=u1 < 125  ElseIfExpressions=u1 > 125 & u1 < 175, u1 > 175  ShowElse=off
  If Action Subsystem : Subsystem  TreatAsAtomicUnit=on
  If Action Subsystem1 : Subsystem  TreatAsAtomicUnit=on
  If Action Subsystem2 : Subsystem  TreatAsAtomicUnit=on
  Merge : Merge  Inputs=3
  Saturation2 : Saturate  UpperLimit=1  LowerLimit=0
  Scope : Scope
      settings: ActiveDisplayYMinimum=0.9  ActiveDisplayYMaximum=1.1  DataLoggingVariableName=ScopeData2
  derate_pos : Outport
  derate_neg : Outport  Port=2
  wires:
  If/1 -> If Action Subsystem/Action
  Tj/1 -> If/1, If Action Subsystem1/1(Tj)
  If/3 -> If Action Subsystem2/Action
  If/2 -> If Action Subsystem1/Action
  If Action Subsystem2/1(Out1) -> Merge/3
  If Action Subsystem1/1(Out1) -> Merge/2
  Merge/1 -> Saturation2/1
  If Action Subsystem/1(Out1) -> Merge/1
  Gain2/1 -> derate_pos/1, Gain/1
  Saturation2/1 -> Scope/1, Gain2/1  "DAB_EF_derate_factor"
  Gain/1 -> derate_neg/1

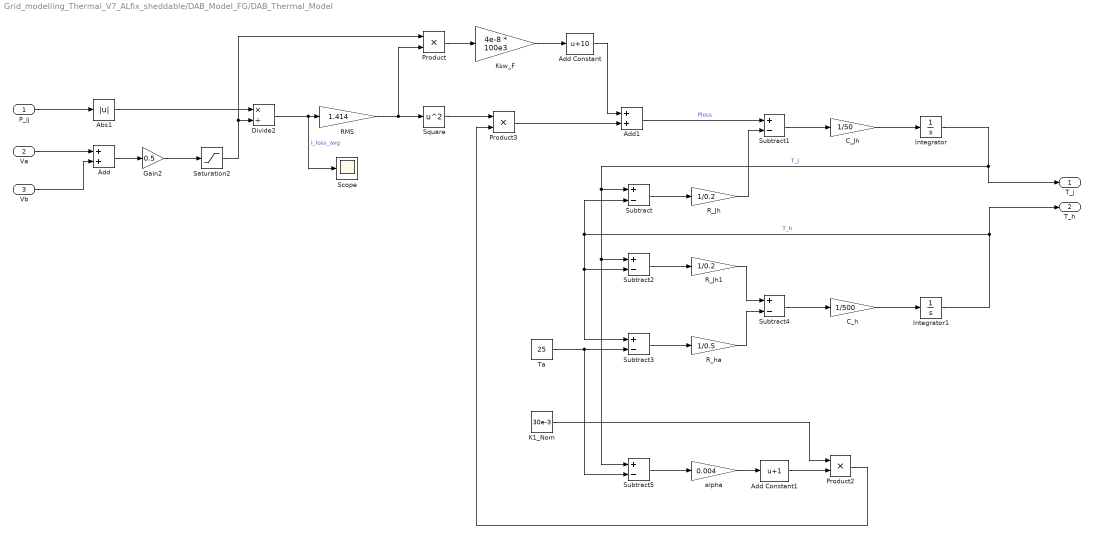
== system Grid_modelling_Thermal_V7_ALfix_sheddable/DAB_Model_FG/DAB_Thermal_Model ==
  P_ij : Inport
  Va : Inport  Port=2
  Vb : Inport  Port=3
  Abs1 : Abs  SaturateOnIntegerOverflow=off
  Add : Sum
  Add Constant : Bias  Bias=10  SaturateOnIntegerOverflow=off
  Add Constant1 : Bias  Bias=1  SaturateOnIntegerOverflow=off
  Add1 : Sum
  C_Jh : Gain  Gain=1/50
  C_h : Gain  Gain=1/500
  Divide2 : Product  Inputs=*/
  Gain2 : Gain  Gain=0.5
  Integrator : Integrator  InitialCondition=25
  Integrator1 : Integrator  InitialCondition=25
  K1_Nom : Constant  Value=30e-3
  Ksw_F : Gain  Gain=4e-8 * 100e3
  Product : Product
  Product2 : Product
  Product3 : Product
  RMS : Gain  Gain=1.414
  R_Jh : Gain  Gain=1/0.2
  R_Jh1 : Gain  Gain=1/0.2
  R_ha : Gain  Gain=1/0.5
  Saturation2 : Saturate  UpperLimit=inf  LowerLimit=1e-3
  Scope : Scope
      settings: ActiveDisplayYMinimum=-5.76507  ActiveDisplayYMaximum=51.88567
  Square : Math  Operator=square
  Subtract{,1..5} (6 alike) : Sum  Inputs=+-
  Ta : Constant  Value=25
  alpha : Gain  Gain=0.004
  T_j : Outport
  T_h : Outport  Port=2
  wires:
  Integrator/1 -> T_j/1, Subtract5/1, Subtract2/1, Subtract/1  "T_j"
  Add1/1 -> Subtract1/1  "Ploss"
  R_ha/1 -> Subtract4/2
  Gain2/1 -> Saturation2/1
  Va/1 -> Add/1
  Integrator1/1 -> T_h/1, Subtract/2, Subtract3/1, Subtract2/2  "T_h"
  R_Jh/1 -> Subtract1/2
  Add/1 -> Gain2/1
  Subtract5/1 -> alpha/1
  Subtract1/1 -> C_Jh/1
  C_h/1 -> Integrator1/1
  Divide2/1 -> Scope/1, RMS/1  "I_loss_avg"
  Product3/1 -> Add1/2
  P_ij/1 -> Abs1/1
  Subtract2/1 -> R_Jh1/1
  alpha/1 -> Add Constant1/1
  Product2/1 -> Product3/2
  C_Jh/1 -> Integrator/1
  Ta/1 -> Subtract5/2, Subtract3/2
  Saturation2/1 -> Product/1, Divide2/2
  R_Jh1/1 -> Subtract4/1
  Subtract/1 -> R_Jh/1
  Abs1/1 -> Divide2/1
  Subtract4/1 -> C_h/1
  Subtract3/1 -> R_ha/1
  Add Constant1/1 -> Product2/2
  Vb/1 -> Add/2
  K1_Nom/1 -> Product2/1
  Square/1 -> Product3/1
  RMS/1 -> Product/2, Square/1
  Product/1 -> Ksw_F/1
  Ksw_F/1 -> Add Constant/1
  Add Constant/1 -> Add1/1

== system Grid_modelling_Thermal_V7_ALfix_sheddable/DAB_Model_FG/thermal_derater ==
  Tj : Inport
  Gain : Gain  Gain=-1
  Gain2 : Gain  Gain=100e3
  If : If  IfExpression=u1 < 125  ElseIfExpressions=u1 > 125 & u1 < 175, u1 > 175  ShowElse=off
  If Action Subsystem : Subsystem  TreatAsAtomicUnit=on
  If Action Subsystem1 : Subsystem  TreatAsAtomicUnit=on
  If Action Subsystem2 : Subsystem  TreatAsAtomicUnit=on
  Merge : Merge  Inputs=3
  Saturation2 : Saturate  UpperLimit=1  LowerLimit=0
  Scope : Scope
      settings: ActiveDisplayYMinimum=0.11326  ActiveDisplayYMaximum=1.09853  DataLoggingVariableName=ScopeData2
  derate_pos : Outport
  derate_neg : Outport  Port=2
  wires:
  If/1 -> If Action Subsystem/Action
  Tj/1 -> If/1, If Action Subsystem1/1(Tj)
  If/3 -> If Action Subsystem2/Action
  If/2 -> If Action Subsystem1/Action
  If Action Subsystem2/1(Out1) -> Merge/3
  If Action Subsystem1/1(Out1) -> Merge/2
  Merge/1 -> Saturation2/1
  If Action Subsystem/1(Out1) -> Merge/1
  Gain2/1 -> derate_pos/1, Gain/1
  Saturation2/1 -> Scope/1, Gain2/1  "DAB_FG_derate_factor"
  Gain/1 -> derate_neg/1

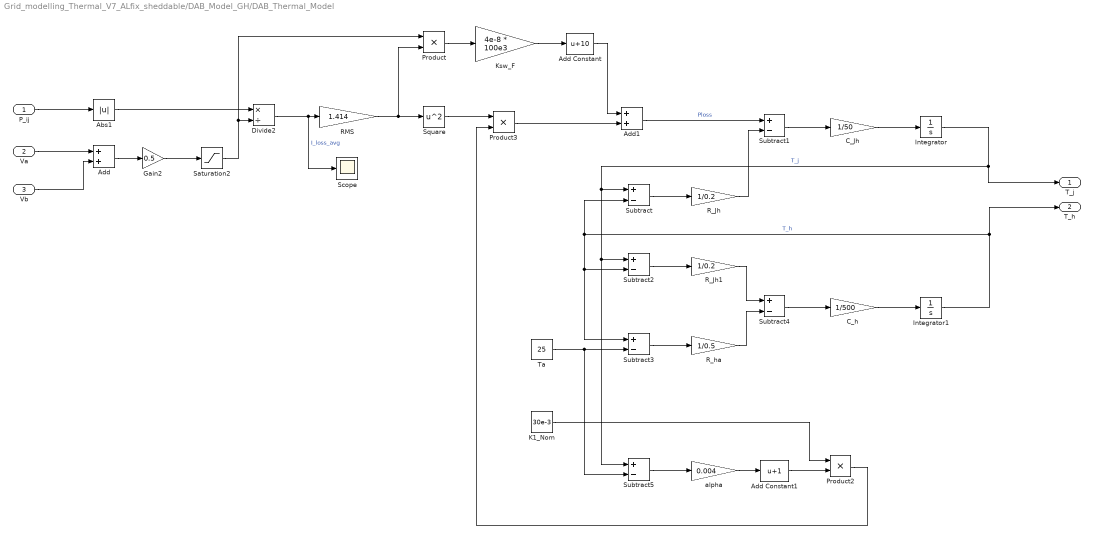
== system Grid_modelling_Thermal_V7_ALfix_sheddable/DAB_Model_GH/DAB_Thermal_Model ==
  P_ij : Inport
  Va : Inport  Port=2
  Vb : Inport  Port=3
  Abs1 : Abs  SaturateOnIntegerOverflow=off
  Add : Sum
  Add Constant : Bias  Bias=10  SaturateOnIntegerOverflow=off
  Add Constant1 : Bias  Bias=1  SaturateOnIntegerOverflow=off
  Add1 : Sum
  C_Jh : Gain  Gain=1/50
  C_h : Gain  Gain=1/500
  Divide2 : Product  Inputs=*/
  Gain2 : Gain  Gain=0.5
  Integrator : Integrator  InitialCondition=25
  Integrator1 : Integrator  InitialCondition=25
  K1_Nom : Constant  Value=30e-3
  Ksw_F : Gain  Gain=4e-8 * 100e3
  Product : Product
  Product2 : Product
  Product3 : Product
  RMS : Gain  Gain=1.414
  R_Jh : Gain  Gain=1/0.2
  R_Jh1 : Gain  Gain=1/0.2
  R_ha : Gain  Gain=1/0.5
  Saturation2 : Saturate  UpperLimit=inf  LowerLimit=1e-3
  Scope : Scope
      settings: ActiveDisplayYMinimum=-2.45667  ActiveDisplayYMaximum=22.11007
  Square : Math  Operator=square
  Subtract{,1..5} (6 alike) : Sum  Inputs=+-
  Ta : Constant  Value=25
  alpha : Gain  Gain=0.004
  T_j : Outport
  T_h : Outport  Port=2
  wires:
  Integrator/1 -> T_j/1, Subtract5/1, Subtract2/1, Subtract/1  "T_j"
  Add1/1 -> Subtract1/1  "Ploss"
  R_ha/1 -> Subtract4/2
  Gain2/1 -> Saturation2/1
  Va/1 -> Add/1
  Integrator1/1 -> T_h/1, Subtract/2, Subtract3/1, Subtract2/2  "T_h"
  R_Jh/1 -> Subtract1/2
  Add/1 -> Gain2/1
  Subtract5/1 -> alpha/1
  Subtract1/1 -> C_Jh/1
  C_h/1 -> Integrator1/1
  Divide2/1 -> Scope/1, RMS/1  "I_loss_avg"
  Product3/1 -> Add1/2
  P_ij/1 -> Abs1/1
  Subtract2/1 -> R_Jh1/1
  alpha/1 -> Add Constant1/1
  Product2/1 -> Product3/2
  C_Jh/1 -> Integrator/1
  Ta/1 -> Subtract5/2, Subtract3/2
  Saturation2/1 -> Product/1, Divide2/2
  R_Jh1/1 -> Subtract4/1
  Subtract/1 -> R_Jh/1
  Abs1/1 -> Divide2/1
  Subtract4/1 -> C_h/1
  Subtract3/1 -> R_ha/1
  Add Constant1/1 -> Product2/2
  Vb/1 -> Add/2
  K1_Nom/1 -> Product2/1
  Square/1 -> Product3/1
  RMS/1 -> Product/2, Square/1
  Product/1 -> Ksw_F/1
  Ksw_F/1 -> Add Constant/1
  Add Constant/1 -> Add1/1

== system Grid_modelling_Thermal_V7_ALfix_sheddable/DAB_Model_GH/thermal_derater ==
  Tj : Inport
  Gain : Gain  Gain=-1
  Gain2 : Gain  Gain=100e3
  If : If  IfExpression=u1 < 125  ElseIfExpressions=u1 > 125 & u1 < 175, u1 > 175  ShowElse=off
  If Action Subsystem : Subsystem  TreatAsAtomicUnit=on
  If Action Subsystem1 : Subsystem  TreatAsAtomicUnit=on
  If Action Subsystem2 : Subsystem  TreatAsAtomicUnit=on
  Merge : Merge  Inputs=3
  Saturation2 : Saturate  UpperLimit=1  LowerLimit=0
  Scope : Scope
      settings: ActiveDisplayYMinimum=0.9  ActiveDisplayYMaximum=1.1  DataLoggingVariableName=ScopeData2
  derate_pos : Outport
  derate_neg : Outport  Port=2
  wires:
  If/1 -> If Action Subsystem/Action
  Tj/1 -> If/1, If Action Subsystem1/1(Tj)
  If/3 -> If Action Subsystem2/Action
  If/2 -> If Action Subsystem1/Action
  If Action Subsystem2/1(Out1) -> Merge/3
  If Action Subsystem1/1(Out1) -> Merge/2
  Merge/1 -> Saturation2/1
  If Action Subsystem/1(Out1) -> Merge/1
  Gain2/1 -> derate_pos/1, Gain/1
  Saturation2/1 -> Scope/1, Gain2/1  "DAB_GH_derate_factor"
  Gain/1 -> derate_neg/1

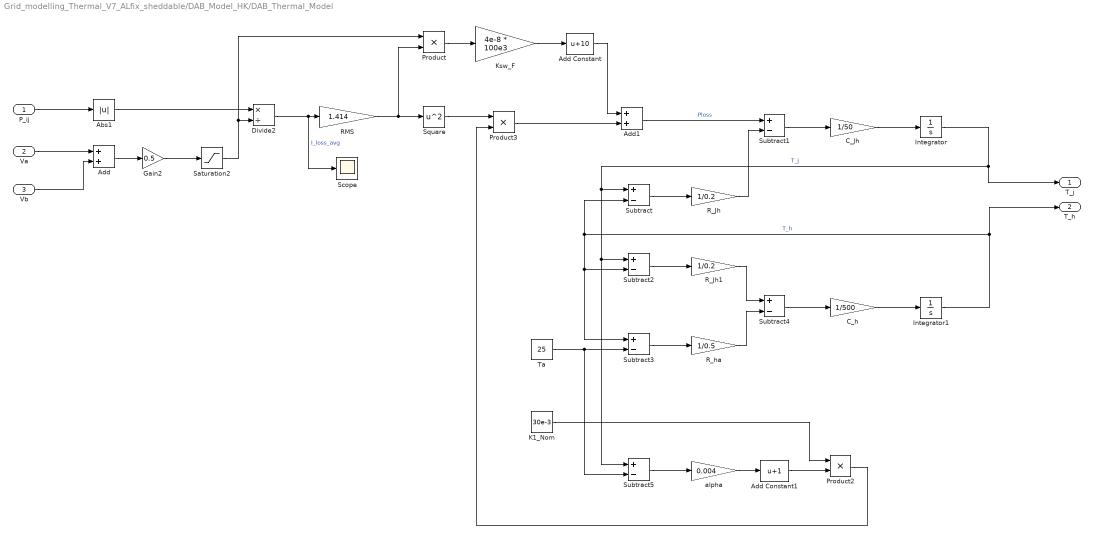
== system Grid_modelling_Thermal_V7_ALfix_sheddable/DAB_Model_HK/DAB_Thermal_Model ==
  P_ij : Inport
  Va : Inport  Port=2
  Vb : Inport  Port=3
  Abs1 : Abs  SaturateOnIntegerOverflow=off
  Add : Sum
  Add Constant : Bias  Bias=10  SaturateOnIntegerOverflow=off
  Add Constant1 : Bias  Bias=1  SaturateOnIntegerOverflow=off
  Add1 : Sum
  C_Jh : Gain  Gain=1/50
  C_h : Gain  Gain=1/500
  Divide2 : Product  Inputs=*/
  Gain2 : Gain  Gain=0.5
  Integrator : Integrator  InitialCondition=25
  Integrator1 : Integrator  InitialCondition=25
  K1_Nom : Constant  Value=30e-3
  Ksw_F : Gain  Gain=4e-8 * 100e3
  Product : Product
  Product2 : Product
  Product3 : Product
  RMS : Gain  Gain=1.414
  R_Jh : Gain  Gain=1/0.2
  R_Jh1 : Gain  Gain=1/0.2
  R_ha : Gain  Gain=1/0.5
  Saturation2 : Saturate  UpperLimit=inf  LowerLimit=1e-3
  Scope : Scope
      settings: ActiveDisplayYMinimum=-2.45667  ActiveDisplayYMaximum=22.11007
  Square : Math  Operator=square
  Subtract{,1..5} (6 alike) : Sum  Inputs=+-
  Ta : Constant  Value=25
  alpha : Gain  Gain=0.004
  T_j : Outport
  T_h : Outport  Port=2
  wires:
  Integrator/1 -> T_j/1, Subtract5/1, Subtract2/1, Subtract/1  "T_j"
  Add1/1 -> Subtract1/1  "Ploss"
  R_ha/1 -> Subtract4/2
  Gain2/1 -> Saturation2/1
  Va/1 -> Add/1
  Integrator1/1 -> T_h/1, Subtract/2, Subtract3/1, Subtract2/2  "T_h"
  R_Jh/1 -> Subtract1/2
  Add/1 -> Gain2/1
  Subtract5/1 -> alpha/1
  Subtract1/1 -> C_Jh/1
  C_h/1 -> Integrator1/1
  Divide2/1 -> Scope/1, RMS/1  "I_loss_avg"
  Product3/1 -> Add1/2
  P_ij/1 -> Abs1/1
  Subtract2/1 -> R_Jh1/1
  alpha/1 -> Add Constant1/1
  Product2/1 -> Product3/2
  C_Jh/1 -> Integrator/1
  Ta/1 -> Subtract5/2, Subtract3/2
  Saturation2/1 -> Product/1, Divide2/2
  R_Jh1/1 -> Subtract4/1
  Subtract/1 -> R_Jh/1
  Abs1/1 -> Divide2/1
  Subtract4/1 -> C_h/1
  Subtract3/1 -> R_ha/1
  Add Constant1/1 -> Product2/2
  Vb/1 -> Add/2
  K1_Nom/1 -> Product2/1
  Square/1 -> Product3/1
  RMS/1 -> Product/2, Square/1
  Product/1 -> Ksw_F/1
  Ksw_F/1 -> Add Constant/1
  Add Constant/1 -> Add1/1

== system Grid_modelling_Thermal_V7_ALfix_sheddable/DAB_Model_HK/thermal_derater ==
  Tj : Inport
  Gain : Gain  Gain=-1
  Gain2 : Gain  Gain=100e3
  If : If  IfExpression=u1 < 125  ElseIfExpressions=u1 > 125 & u1 < 175, u1 > 175  ShowElse=off
  If Action Subsystem : Subsystem  TreatAsAtomicUnit=on
  If Action Subsystem1 : Subsystem  TreatAsAtomicUnit=on
  If Action Subsystem2 : Subsystem  TreatAsAtomicUnit=on
  Merge : Merge  Inputs=3
  Saturation2 : Saturate  UpperLimit=1  LowerLimit=0
  Scope : Scope
      settings: ActiveDisplayYMinimum=0.11289  ActiveDisplayYMaximum=1.09857  DataLoggingVariableName=ScopeData2
  derate_pos : Outport
  derate_neg : Outport  Port=2
  wires:
  If/1 -> If Action Subsystem/Action
  Tj/1 -> If/1, If Action Subsystem1/1(Tj)
  If/3 -> If Action Subsystem2/Action
  If/2 -> If Action Subsystem1/Action
  If Action Subsystem2/1(Out1) -> Merge/3
  If Action Subsystem1/1(Out1) -> Merge/2
  Merge/1 -> Saturation2/1
  If Action Subsystem/1(Out1) -> Merge/1
  Gain2/1 -> derate_pos/1, Gain/1
  Saturation2/1 -> Scope/1, Gain2/1  "DAB_HK_derate_factor"
  Gain/1 -> derate_neg/1
